simulink model "Solarpannel"  (R2021a)
settings: Solver=VariableStepAuto  StartTime=0.0  StopTime=10.0  RelTol=1e-3
libraries: spsDiodeLib x7, spsMosfetLib x6, spsSeriesRLCBranchLib x5, spsVoltageMeasurementLib x3, spsThreePhaseVIMeasurementLib x2, spspowerguiLib x2, spsCurrentMeasurementLib x1, spsDCVoltageSourceLib x1, spsGroundLib x1, spsIGBTLib x1, simulink x1, spsPVArrayLib x1
settings Model: Creator=Harshitha  LastModifiedBy=Harshitha

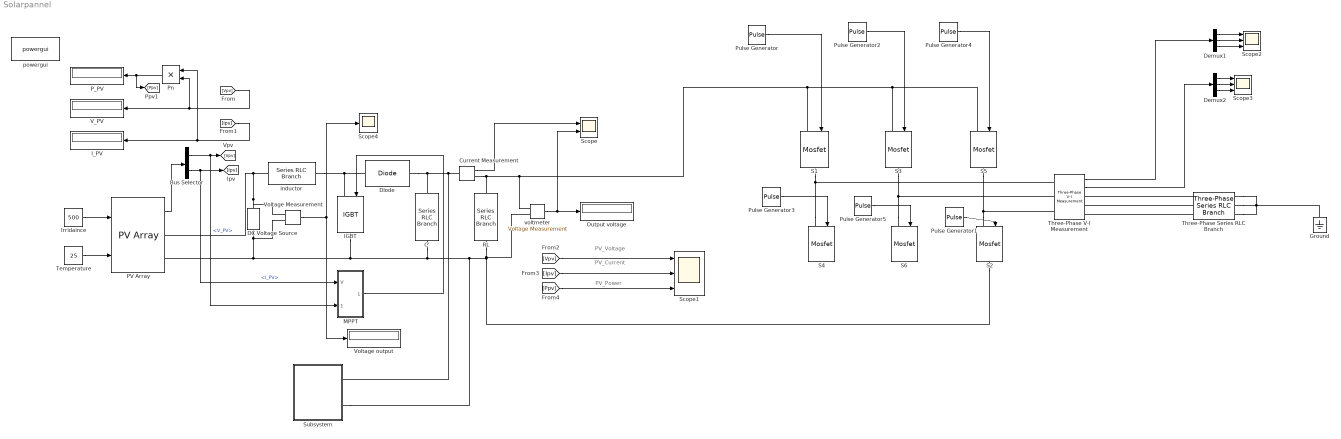
== system Solarpannel ==
  note: PV_Power
  note: PV_Current
  note: PV_Voltage
  Bus Selector : BusSelector  OutputSignals=V_PV,I_PV
  C' : spsSeriesRLCBranchLib/Series RLC Branch  LConnTagsString=__new0  RConnTagsString=__new0  BranchType=C  Resistance=1  Inductance=1e-3  SetiL0=off  InitialCurrent=0  Capacitance=25e-6  Setx0=off  InitialVoltage=0  Measurements=None
  Current Measurement : spsCurrentMeasurementLib/Current Measurement  PhasorSimulation=off  OutputType=Complex  PSBequivalent=0
  DC Voltage Source : spsDCVoltageSourceLib/DC Voltage Source  Amplitude=100  Measurements=None
  Demux1 : Demux  Outputs=3
  Demux2 : Demux  Outputs=3
  Diode : spsDiodeLib/Diode  Ron=0.001  Lon=0  Vf=0.8  IC=0  UseSnubber=0  Rs=500  Cs=250e-9  Measurements=off
  Ground : spsGroundLib/Ground  LConnTagsString=a
  IGBT : spsIGBTLib/IGBT  Ron=0.001  Lon=0  Vf=1  Tf=1e-6  Tt=2e-6  IC=0  Rs=1e5  Cs=inf  Measurements=off
  I_PV : Display
  Irridaince : Constant  Value=500
  MPPT : Subsystem
  Output voltage : Display
  PV Array : spsPVArrayLib/PV Array  Npar=4  Nser=10  PlotType=array @ 25 deg.C & specified irradiances  S_vec=[800 500 ]  Temp_C_vec=[800 500]  ModuleName=Trina Solar TSM-250PA05.08  PlotWhenSelected=off  Pm=249.86  Ncell=60  Voc=37.6  Isc=8.55  Vm=31  Im=8.06  beta_Voc_pc=-0.35  alpha_Isc_pc=0.06  beta_Voc=-0.1316  alpha_Isc=0.00513  IL=8.5795  I0=2.0381e-10  nI=0.99766  Rsh=301.8149  Rs=0.247  RobustModel=off  RobustCellTemperature=313.3991  BAL=on  Tc=1e-6  Tfilter=5e-5
  P_PV : Display
  Pn : Product
  Pulse Generator : DiscretePulseGenerator  PulseType=Time based  Period=0.02  PulseWidth=50
  Pulse Generator1 : DiscretePulseGenerator  PulseType=Time based  Period=0.02  PulseWidth=50  PhaseDelay=(3.33e-3)*1
  Pulse Generator2 : DiscretePulseGenerator  PulseType=Time based  Period=0.02  PulseWidth=50  PhaseDelay=(3.33e-3)*2
  Pulse Generator3 : DiscretePulseGenerator  PulseType=Time based  Period=0.02  PulseWidth=50  PhaseDelay=(3.33e-3)*3
  Pulse Generator4 : DiscretePulseGenerator  PulseType=Time based  Period=0.02  PulseWidth=50  PhaseDelay=(3.33e-3)*4
  Pulse Generator5 : DiscretePulseGenerator  PulseType=Time based  Period=0.02  PulseWidth=50  PhaseDelay=(3.33e-3)*5
  RL : spsSeriesRLCBranchLib/Series RLC Branch  LConnTagsString=__new0  RConnTagsString=__new0  BranchType=R  Resistance=10  Inductance=1e-3  SetiL0=off  InitialCurrent=0  Capacitance=1e-6  Setx0=off  InitialVoltage=0  Measurements=None
  S{1..6} (6 alike) : spsMosfetLib/Mosfet  Ron=0.1  Lon=0  Rd=0.01  Vfd=0  IC=0  Rs=1e5  Cs=inf  Measurements=off
  Scope : Scope  NumInputPorts=2
  Scope1 : Scope  NumInputPorts=3
  Scope2 : Scope  NumInputPorts=3
  Scope3 : Scope  NumInputPorts=3
  Scope4 : Scope
  Subsystem : Subsystem
  Temperature : Constant  Value=25
  Three-Phase Series RLC Branch : spsThreePhaseSeriesRLCBranchLib/Three-Phase Series RLC Branch  LConnTagsString=A|B|C  RConnTagsString=A|B|C  BranchType=R  Resistance=100  Inductance=1e-3  Capacitance=1e-6  Measurements=None
  Three-Phase V-I Measurement : spsThreePhaseVIMeasurementLib/Three-Phase V-I Measurement  VoltageMeasurement=phase-to-ground  SetLabelV=off  LabelV=Vabc  Vpu=off  VpuLL=off  CurrentMeasurement=yes  SetLabelI=off  LabelI=Iabc  Ipu=off  Pbase=100e6  Vbase=500e3  OutputType=Complex  PhasorSimulation=off  PSBequivalent=0
  V_PV : Display
  Voltage Measurement : spsVoltageMeasurementLib/Voltage Measurement  PhasorSimulation=off  OutputType=Complex  PSBequivalent=0
  Voltage output : Display
  inductor : spsSeriesRLCBranchLib/Series RLC Branch  LConnTagsString=__new0  RConnTagsString=__new0  BranchType=L  Resistance=1  Inductance=19.53e-6  SetiL0=off  InitialCurrent=0  Capacitance=1e-6  Setx0=off  InitialVoltage=0  Measurements=None
  powergui : spspowerguiLib/powergui  Priority=1  SimulationMode=Discrete  SampleTime=50e-6  frequency=60  Iterations=50  frequencyindice=0  Pbase=100e6  ErrMax=1e-4  UnitsV=kV  UnitsW=MW  buscounter=0  FunctionMessages=off  echomessages=off  EnableUseOfTLC=off  CurrentSourceSwitches=off  DisableSnubberDevices=off  DisableRonSwitches=off  DisableVfSwitches=off  DisplayEquations=off  AutomaticDiscreteSolvers=off  SolverType=Tustin/Backward Euler (TBE)  Interpol=off  ExternalGateDelay=off  methode=off  Ts=100  x0status=blocks  SPID=on  SwTol=0  HookPort=off  NonlinearTolerance=1e-4  nMaxIteration=100  ContinueOnMaxIteration=off  RestoreLinks=warning  ResistiveCurrentMeasurement=off  Frange=[0:2:500]  Ylog=off  Xlog=on  ShowGrid=off  save=off  variable=ZData  structure=0  ZoomFFT=off  StartTime=0.0  cycles=1  DisplayStyle=1  fundamental=60  FreqAxis=off  MaxFrequency=1000  frequencyindicesteady=1  RmsSteady=1  display=off
  voltmeter : spsVoltageMeasurementLib/Voltage Measurement  PhasorSimulation=off  OutputType=Complex  PSBequivalent=0
  wires:
  Irridaince/1 -> PV Array/1
  Temperature/1 -> PV Array/2
  voltmeter/1 -> Scope/2, Output voltage/1
  PV Array/1 -> Bus Selector/1
  Bus Selector/2 -> MPPT/1(V), [Ipv]  "<I_PV>"
  Bus Selector/1 -> MPPT/2(1), [Vpv]  "<V_PV>"
  Current Measurement/1 -> Scope/1
  Pn/1 -> [Ppv], P_PV/1
  [Vpv] -> V_PV/1, Pn/2
  [Ipv] -> Pn/1, I_PV/1
  [Vpv] -> Scope1/1
  [Ipv] -> Scope1/2
  [Ppv] -> Scope1/3
  Three-Phase V-I Measurement/2 -> Demux2/1
  Pulse Generator1/1 -> S2/1
  Pulse Generator5/1 -> S6/1
  Pulse Generator2/1 -> S3/1
  Demux2/2 -> Scope3/2
  Pulse Generator4/1 -> S5/1
  Demux2/1 -> Scope3/1
  Pulse Generator/1 -> S1/1
  Demux1/1 -> Scope2/1
  Pulse Generator3/1 -> S4/1
  Demux2/3 -> Scope3/3
  Three-Phase V-I Measurement/1 -> Demux1/1
  Demux1/3 -> Scope2/3
  Demux1/2 -> Scope2/2
  Voltage Measurement/1 -> Scope4/1, Voltage output/1
  MPPT/1(Out2) -> IGBT/1
  connections:
  Current Measurement/LConn1 -- C'/LConn1 -- Diode/RConn1 -- Subsystem/RConn1
  IGBT/LConn1 -- Diode/LConn1 -- inductor/RConn1
  Current Measurement/RConn1 -- voltmeter/LConn1 -- S1/LConn1 -- S3/LConn1 -- S5/LConn1 -- RL/LConn1
  DC Voltage Source/RConn1 -- inductor/LConn1 -- PV Array/RConn1 -- Voltage Measurement/LConn1
  S4/LConn1 -- S1/RConn1 -- Three-Phase V-I Measurement/LConn1
  Three-Phase Series RLC Branch/RConn1 -- Three-Phase Series RLC Branch/RConn2 -- Ground/LConn1 -- Three-Phase Series RLC Branch/RConn3
  S2/LConn1 -- S5/RConn1 -- Three-Phase V-I Measurement/LConn3
  S6/LConn1 -- S3/RConn1 -- Three-Phase V-I Measurement/LConn2
  Three-Phase Series RLC Branch/LConn1 -- Three-Phase V-I Measurement/RConn1
  Three-Phase Series RLC Branch/LConn3 -- Three-Phase V-I Measurement/RConn3
  Three-Phase Series RLC Branch/LConn2 -- Three-Phase V-I Measurement/RConn2
  C'/RConn1 -- Subsystem/RConn2 -- S2/RConn1 -- voltmeter/LConn2 -- RL/RConn1 -- IGBT/RConn1 -- Voltage Measurement/LConn2 -- DC Voltage Source/LConn1 -- PV Array/RConn2

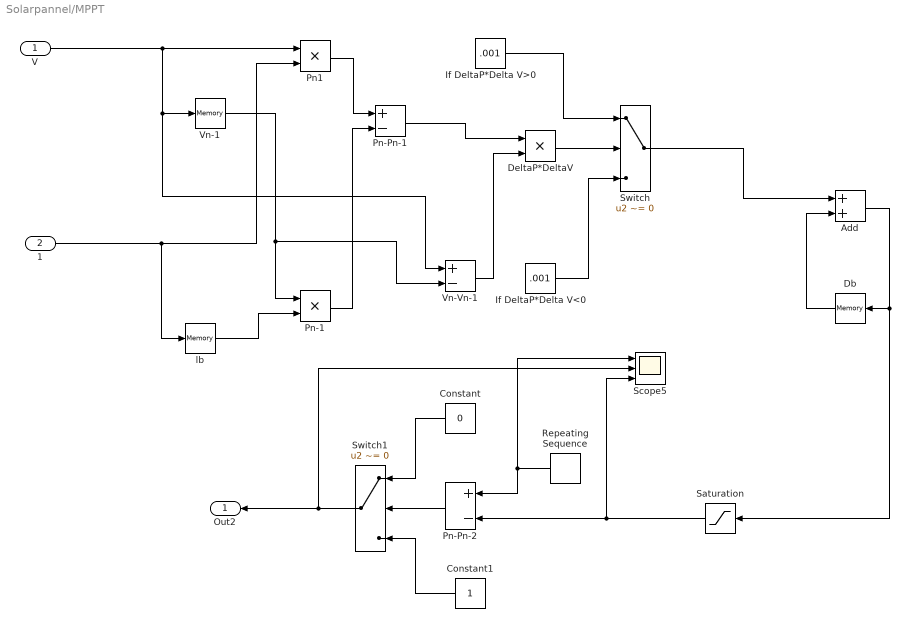
== system Solarpannel/MPPT ==
  V : Inport
  1 : Inport  Port=2
  Add : Sum
  Constant : Constant  Value=0
  Constant1 : Constant
  Db : Memory  LinearizeAsDelay=on
  DeltaP*DeltaV : Product
  If DeltaP*Delta V<0 : Constant  Value=.001
  If DeltaP*Delta V>0 : Constant  Value=.001
  Pn-1 : Product
  Pn-Pn-1 : Sum  Inputs=+-
  Pn-Pn-2 : Sum  Inputs=+-
  Pn1 : Product
  Repeating Sequence : simulink/Sources/Repeating Sequence  rep_seq_t=[0 4e-4]  rep_seq_y=[0 1]
  Saturation : Saturate  UpperLimit=1
  Scope5 : Scope  NumInputPorts=3
  Switch : Switch  Criteria=u2 ~= 0  ZeroCross=off
  Switch1 : Switch  Criteria=u2 ~= 0
  Vn-1 : Memory
  Vn-Vn-1 : Sum  Inputs=+-
  lb : Memory
  Out2 : Outport
  wires:
  Repeating Sequence/1 -> Pn-Pn-2/1, Scope5/1
  Add/1 -> Db/1, Saturation/1
  lb/1 -> Pn-1/2
  Switch1/1 -> Out2/1, Scope5/2
  Pn-Pn-1/1 -> DeltaP*DeltaV/1
  If DeltaP*Delta V>0/1 -> Switch/1
  Constant1/1 -> Switch1/3
  1/1 -> Pn1/2, lb/1
  Saturation/1 -> Scope5/3, Pn-Pn-2/2
  V/1 -> Pn1/1, Vn-Vn-1/1, Vn-1/1
  Pn-Pn-2/1 -> Switch1/2
  Vn-1/1 -> Pn-1/1, Vn-Vn-1/2
  Db/1 -> Add/2
  Constant/1 -> Switch1/1
  If DeltaP*Delta V<0/1 -> Switch/3
  Pn1/1 -> Pn-Pn-1/1
  Vn-Vn-1/1 -> DeltaP*DeltaV/2
  DeltaP*DeltaV/1 -> Switch/2
  Pn-1/1 -> Pn-Pn-1/2
  Switch/1 -> Add/1

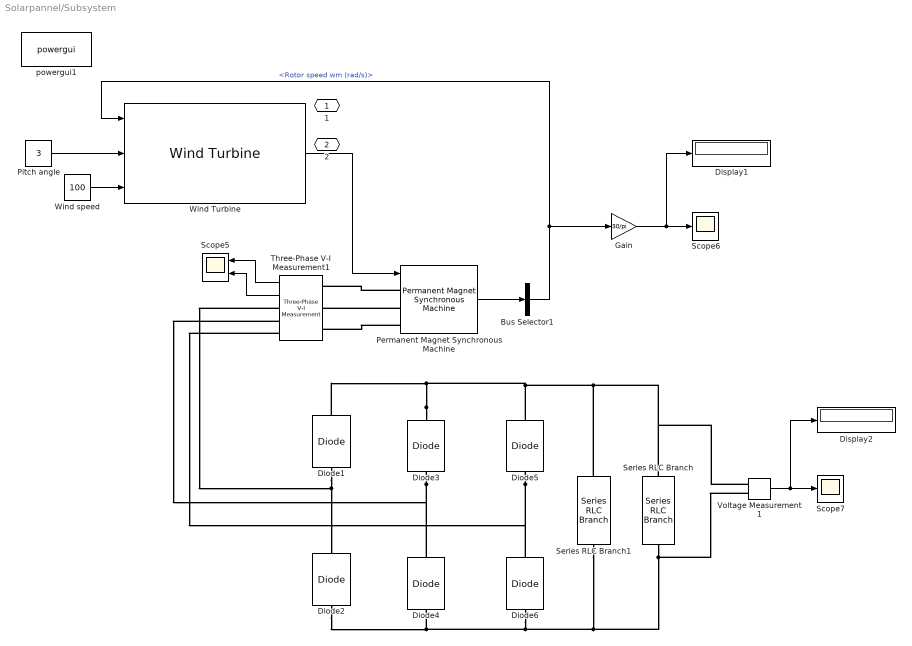
== system Solarpannel/Subsystem ==
  Bus Selector1 : BusSelector  OutputSignals=Rotor speed wm (rad/s)
  Diode{1..6} (6 alike) : spsDiodeLib/Diode  Ron=0.001  Lon=0  Vf=0.8  IC=0  UseSnubber=0  Rs=500  Cs=250e-9  Measurements=off
  Display1 : Display
  Display2 : Display
  Gain : Gain  Gain=30/pi
  Permanent Magnet Synchronous Machine : spsPermanentMagnetSynchronousMachineLib/Permanent Magnet Synchronous Machine  NbPhases=3  FluxDistribution=Sinusoidal  RotorType=Round  MechanicalLoad=Torque Tm  PresetModel=No  ShowDetailedParameters=on  MeasurementBus=off  Resistance=0.0485  Inductance=8.5e-3  dqInductances=[8.5e-3,8.5e-3]  La=0.000395  MachineConstant=Flux linkage established by magnets (V.s)  Flux=0.1194  VoltageCst=86.6271  TorqueCst=0.7164  Flat=120  Mechanical=[0.0027 0.0004924 4 0]  PolePairs=4  InitialConditions=[0,0, 0,0]  InitialConditions5ph=[0 0 0 0 0 0]  RefAngle=90 degrees behind phase A axis (modified Park)  IterativeDiscreteModel=Trapezoidal non iterative  TsBlock=-1  TsPowergui=0
  Pitch angle : Constant  Value=3
  Scope5 : Scope  NumInputPorts=2
  Scope6 : Scope
  Scope7 : Scope
  Series RLC Branch : spsSeriesRLCBranchLib/Series RLC Branch  LConnTagsString=__new0  RConnTagsString=__new0  BranchType=R  Resistance=10  Inductance=1e-3  SetiL0=off  InitialCurrent=0  Capacitance=1e-6  Setx0=off  InitialVoltage=0  Measurements=None
  Series RLC Branch1 : spsSeriesRLCBranchLib/Series RLC Branch  LConnTagsString=__new0  RConnTagsString=__new0  BranchType=C  Resistance=1  Inductance=1e-3  SetiL0=off  InitialCurrent=0  Capacitance=10e-3  Setx0=off  InitialVoltage=0  Measurements=None
  Three-Phase V-I Measurement1 : spsThreePhaseVIMeasurementLib/Three-Phase V-I Measurement  VoltageMeasurement=phase-to-phase  SetLabelV=off  LabelV=Vabc  Vpu=off  VpuLL=off  CurrentMeasurement=yes  SetLabelI=off  LabelI=Iabc  Ipu=off  Pbase=100e6  Vbase=500e3  OutputType=Complex  PhasorSimulation=off  PSBequivalent=0
  Voltage Measurement1 : spsVoltageMeasurementLib/Voltage Measurement  PhasorSimulation=off  OutputType=Complex  PSBequivalent=0
  Wind Turbine : spsWindTurbineLib/Wind Turbine  Pnom=1.5e6  Pelec_base=1.5e6/0.9  wind_base=12  P_wind_base=0.73  speed_nom=1.2  pitch_angle=0  c1_c6="[0.51763          116          0.4            5           21     0.006795]"  cp_nom=0.48  lambda_nom=8.1
      settings: SourceProductBaseCode=PS
  Wind speed : Constant  Value=100
  powergui1 : spspowerguiLib/powergui  Priority=1  SimulationMode=Discrete  SampleTime=50e-6  frequency=60  Iterations=50  frequencyindice=0  Pbase=100e6  ErrMax=1e-4  UnitsV=kV  UnitsW=MW  buscounter=0  FunctionMessages=off  echomessages=off  EnableUseOfTLC=off  CurrentSourceSwitches=off  DisableSnubberDevices=off  DisableRonSwitches=off  DisableVfSwitches=off  DisplayEquations=off  AutomaticDiscreteSolvers=off  SolverType=Tustin/Backward Euler (TBE)  Interpol=off  ExternalGateDelay=off  methode=off  Ts=100  x0status=blocks  SPID=on  SwTol=0  HookPort=off  NonlinearTolerance=1e-4  nMaxIteration=100  ContinueOnMaxIteration=off  RestoreLinks=warning  ResistiveCurrentMeasurement=off  Frange=[0:2:500]  Ylog=off  Xlog=on  ShowGrid=off  save=off  variable=ZData  structure=0  ZoomFFT=off  StartTime=0.0  cycles=1  DisplayStyle=1  fundamental=60  FreqAxis=off  MaxFrequency=1000  frequencyindicesteady=1  RmsSteady=1  display=off
  1 : PMIOPort  Side=Right
  2 : PMIOPort  Port=2  Side=Right
  wires:
  Bus Selector1/1 -> Gain/1, Wind Turbine/1  "<Rotor speed wm (rad/s)>"
  Wind speed/1 -> Wind Turbine/3
  Wind Turbine/1 -> Permanent Magnet Synchronous Machine/1
  Permanent Magnet Synchronous Machine/1 -> Bus Selector1/1
  Gain/1 -> Scope6/1, Display1/1
  Voltage Measurement1/1 -> Display2/1, Scope7/1
  Three-Phase V-I Measurement1/1 -> Scope5/1
  Pitch angle/1 -> Wind Turbine/2
  Three-Phase V-I Measurement1/2 -> Scope5/2
  connections:
  Diode5/LConn1 -- Diode6/RConn1 -- Three-Phase V-I Measurement1/RConn3
  Series RLC Branch/RConn1 -- Diode2/LConn1 -- Diode4/LConn1 -- Diode6/LConn1 -- Series RLC Branch1/RConn1 -- Voltage Measurement1/LConn2
  Diode3/RConn1 -- Diode1/RConn1 -- Series RLC Branch1/LConn1 -- Voltage Measurement1/LConn1 -- Series RLC Branch/LConn1 -- Diode5/RConn1
  Diode3/LConn1 -- Diode4/RConn1 -- Three-Phase V-I Measurement1/RConn2
  Three-Phase V-I Measurement1/RConn1 -- Diode1/LConn1 -- Diode2/RConn1
  Permanent Magnet Synchronous Machine/LConn1 -- Three-Phase V-I Measurement1/LConn1
  Permanent Magnet Synchronous Machine/LConn2 -- Three-Phase V-I Measurement1/LConn2
  Permanent Magnet Synchronous Machine/LConn3 -- Three-Phase V-I Measurement1/LConn3
